simulink model "LKAS_AutoSave_DF_20220407_0926_SW62"  (R2018b)
settings: Solver=FixedStepDiscrete  StartTime=0.0  StopTime=10.0  FixedStep=0.01  RelTol=1e-3
InitFcn:
  | tmpVer = ver('MATLAB');
  | tmpVer = str2num(tmpVer.Version);
  | % -------------------------------------------------------------------
  | %  MATLAB file generated by Simulink.saveVars on 21-Nov-2019 10:06:14
  | %  MATLAB version: 7.13.0.564 (R2011b)
  | % -------------------------------------------------------------------
  | 
  | 
  | SInt16 = Simulink.AliasType;
  | SInt16.Description = 'Num';
  | if (tmpVer > 7.11)
  | 	SInt16.DataScope = 'Auto';
  | end
  | SInt16.HeaderFile = 'Rte_Type.h';
  | SInt16.BaseType = 'int16';
  | 
  | SInt32 = Simulink.AliasType;
  | SInt32.Description = 'Num';
  | if (tmpVer > 7.11)
  | 	SInt32.DataScope = 'Auto';
  | end
  | SInt32.HeaderFile = 'Rte_Type.h';
  | SInt32.BaseType = 'int32';
  | 
  | SInt8 = Simulink.AliasType;
  | SInt8.Description = 'Num';
  | if (tmpVer > 7.11)
  | 	SInt8.DataScope = 'Auto';
  | end
  | SInt8.HeaderFile = 'Rte_Type.h';
  | SInt8.BaseType = 'int8';
  | 
  | T_A_m2_1024_1_u32 = Simulink.NumericType;
  | T_A_m2_1024_1_u32.Description = 'm2 (square meters  (m2))';
  | if (tmpVer > 7.11)
  | 	T_A_m2_1024_1_u32.DataScope = 'Auto';
  | end
  | T_A_m2_1024_1_u32.HeaderFile = 'Rte_Type.h';
  | T_A_m2_1024_1_u32.DataTypeMode = 'Fixed-point: slope and bias scaling';
  | T_A_m2_1024_1_u32.SignednessBool = false;
  | T_A_m2_1024_1_u32.WordLength = 32;
  | T_A_m2_1024_1_u32.FixedExponent = -10;
  | T_A_m2_1024_1_u32.SlopeAdjustmentFactor = 1;
  | T_A_m2_1024_1_u32.Bias = 0;
  | T_A_m2_1024_1_u32.DataTypeOverride = 'Inherit';
  | T_A_m2_1024_1_u32.IsAlias = true;
  | 
  | T_A_m2_65536_1_u16 = Simulink.NumericType;
  | T_A_m2_65536_1_u16.Description = 'm2 (square meters  (m2))';
  | if (tmpVer > 7.11)
  | 	T_A_m2_65536_1_u16.DataScope = 'Auto';
  | end
  | T_A_m2_65536_1_u16.HeaderFile = 'Rte_Type.h';
  | T_A_m2_65536_1_u16.DataTypeMode = 'Fixed-point: slope and bias scaling';
  | T_A_m2_65536_1_u16.SignednessBool = false;
  | T_A_m2_65536_1_u16.WordLength = 16;
  | T_A_m2_65536_1_u16.FixedExponent = -16;
  | T_A_m2_65536_1_u16.SlopeAdjustmentFactor = 1;
  | T_A_m2_65536_1_u16.Bias = 0;
  | T_A_m2_65536_1_u16.DataTypeOverride = 'Inherit';
  | ... (+4664 lines)
StopFcn:
  | clear  T_A_m2_1024_1_u32 T_A_m2_65536_1_u16 T_A_m2_Float32 T_A_mm2_10_1_u16 T_A_mm2_4_1_s16 T_A_mm2_Float32 T_Cnt_Num_10_1_u32 T_Cnt_Num_1_1_s16 T_Cnt_Num_1_1_s32 T_Cnt_Num_1_1_s8 T_Cnt_Num_1_1_u16 T_Cnt_Num_1_1_u32 T_Cnt_Num_1_1_u8 T_E_J_1_1_s32 T_E_J_Float32 T_E_kJ_128_1_s32 T_E_kJ_Float32 T_E_kwh_10_1_u16 T_E_kwh_Float32 T_Epl_kwhpkm_100_1_u16 T_Epl_kwhpkm_Float32 T_F_N_1_1_s16 T_F_N_Float32 T_I_A_1000_1_u16 T_I_A_1048576_1_s32 T_I_A_2048_1_s16 T_I_A_32_1_s16 T_I_A_Float32 T_I_mA_1_1_s16 T_I_mA_32768_128_s16 T_I_mA_Float32 T_J_kgpm2_128_1_u16 T_J_kgpm2_Float32 T_K_NA_1000_1_s16 T_K_NA_100_1_s16 T_K_NA_100_1_u16 T_K_NA_1024_1_s16 T_K_NA_1024_1_u16 T_K_NA_128_1_s16 T_K_NA_128_1_u16 T_K_NA_128_1_u8 T_K_NA_16777216_1_u32 T_K_NA_16_1_s16 T_K_NA_16_1_u16 T_K_NA_16_1_u8 T_K_NA_1_16_u16 T_K_NA_1_1_s16 T_K_NA_1_1_u16 T_K_NA_1_1_u8 T_K_NA_32768_1_s16 T_K_NA_32768_1_u16 T_K_NA_32_1_s8 T_K_NA_4096_1_u16 T_K_NA_4194304_1_s32 T_K_NA_4194304_1_u16 T_K_NA_65536_1_s32 T_K_NA_65536_1_u16 T_K_NA_8192_1_s16 T_K_NA_8_1_s16 T_K_NA_Float32 T_M_Nm_16_1_s16 T_M_Nm_1_1_s16 T_M_Nm_32768_1_s16 T_M_Nm_32_1_s16 T_M_Nm_4_1_s16 T_M_Nm_512_1_s16 T_M_Nm_Float32 T_P_W_1_4_s16 T_P_W_1_8_s16 T_P_W_Float32 T_P_kW_128_1_s16 T_P_kW_1_8_s16 T_P_kW_8_1_s32 T_P_kW_Float32 T_Pct_pct_1024_1_s32 T_Pct_pct_1024_1_u32 T_Pct_pct_10_1_s16 T_Pct_pct_10_1_u32 T_Pct_pct_128_100_s8 T_Pct_pct_1_1_s16 T_Pct_pct_1_4_u8 T_Pct_pct_255_100_u16 T_Pct_pct_255_100_u8 T_Pct_pct_256_1_s16 T_Pct_pct_256_1_u16 T_Pct_pct_65535_100_u16 T_Pct_pct_Float32 T_R_ohm_1024_1_s16 T_R_ohm_32_1_s16 T_R_ohm_Float32 T_TK_K_16_1_s16 T_TK_K_Float32 T_T_degC_10_400_1_u16 T_T_degC_16_1_s16 T_T_degC_1_40_1_u8 T_T_degC_2_80_1_u8 T_T_degC_Float32 T_U_V_1000_1_u16 T_U_V_10_1_u8 T_U_V_200_1_u8 T_U_V_32_1_s16 T_U_V_4096_1_s16 T_U_V_512_1_s16 T_U_V_65535_8_u16 T_U_V_8192_1_u16 T_U_V_Float32 T_U_mV_1_1_s16 T_U_mV_256_20_u16 T_U_mV_Float32 T_V_l_256_1_s16 T_V_l_4096_1_s16 T_V_l_64_1_s16 T_V_l_65535_100_u16 T_V_l_Float32 T_V_ml_128_1_s16 T_V_ml_1_1_s16 T_V_ml_32768_1_s16 T_V_ml_Float32 T_V_ul_32_1_u16 T_V_ul_Float32 T_Vpl_clpkm_512_1_u16 T_Vpl_clpkm_Float32 T_a_kphps_16_1_s16 T_a_kphps_Float32 T_a_mps2_128_1_s16 T_a_mps2_Float32 T_c_MJpkg_256_1_s16 T_c_MJpkg_Float32 T_c_kJpgpK_1024_1_s16 T_c_kJpgpK_Float32 T_c_kJpkgpK_128_1_u16 T_c_kJpkgpK_Float32 T_chrg_Ah_1_1_s16 T_chrg_Ah_1_1_u16 T_chrg_Ah_1_1_u8 T_chrg_Ah_256_1_u16 T_chrg_Ah_4194304_1_s32 T_chrg_Ah_512_1_u16 T_chrg_Ah_8_1_u16 T_chrg_Ah_Float32 T_cmp_NA_100_1_s16 T_cmp_NA_128_1_s16 T_cmp_NA_16_1_s16 T_cmp_NA_32768_1_u16 T_cmp_NA_Float32 T_d2n_rpmps2_4_1_s16 T_d2n_rpmps2_Float32 T_dPct_pctps_16_1_s16 T_dPct_pctps_256_1_s16 T_dPct_pctps_Float32 T_dT_degCps_128_1_s16 T_dT_degCps_Float32 T_dV_lph_1_1_s16 T_dV_lph_Float32 T_dV_lpm_128_1_s16 T_dV_lpm_32_1_s16 T_dV_lpm_Float32 T_dV_lps_1024_1_u16 T_dV_lps_4_1_u16 T_dV_lps_Float32 T_dV_mlps_1024_1_s16 T_dV_mlps_Float32 T_d_BitField16 T_dm_gps_128_1_s16 T_dm_gps_128_1_u16 T_dm_gps_256_1_u16 T_dm_gps_Float32 T_dm_mgps_1_1_s16 T_dm_mgps_Float32 T_dn_rpmps_1_1_s16 T_dn_rpmps_2_1_s16 T_dn_rpmps_Float32 T_dp_Paps_1_1_s16 T_dp_Paps_Float32 T_dp_kPaps_1_1_s16 T_dp_kPaps_8_1_s16 T_dp_kPaps_Float32 T_dphi_degps_128_1_s16 T_dphi_degps_8_1_s16 T_dphi_degps_Float32 T_dr_ps_256_1_s16 T_dr_ps_Float32 T_drho_mgplps_1_2_s16 T_drho_mgplps_Float32 T_e_NA_1_1_u8 T_f_Hz_1_1_u16 T_f_Hz_1_1_u32 T_f_Hz_64_1_u16 T_f_Hz_8_1_s16 T_f_Hz_Float32 T_g_BitField32 T_l_km_16_1_s16 T_l_km_1_1_u16 T_l_km_1_1_u32 T_l_km_Float32 T_l_m_1024_1_s16 T_l_m_16_1_s16 T_l_m_1_1_u32 T_l_m_Float32 T_l_mm_16_1_s16 T_l_mm_1_1_u16 T_l_mm_4096_1_s16 T_l_mm_4_1_u8 T_l_mm_64_1_s16 T_l_mm_Float32 T_m_g_1_1_s16 T_m_g_2048_1_s16 T_m_g_32_1_u16 T_m_g_Float32 T_m_kg_1024_1_s16 T_m_kg_1_1_s16 T_m_kg_1_1_u32 T_m_kg_Float32 T_m_mg_128_1_s16 T_m_mg_32_1_s16 T_m_mg_Float32 T_n_rpm_1_1_s16 T_n_rpm_1_25_u8 T_n_rpm_256_50_u16 T_n_rpm_2_25_u8 T_n_rpm_4_1_u16 T_n_rpm_Float32 T_p_MPa_64_1_s16 T_p_MPa_Float32 T_p_Pa_1_1_s16 T_p_Pa_Float32 T_p_kPa_1_10_u16 T_p_kPa_1_1_s16 T_p_kPa_1_1_u8 T_p_kPa_256_1_u16 T_p_kPa_32_1_u16 T_p_kPa_64_1_s16 T_p_kPa_Float32 T_phi_deg_100_1_s16 T_phi_deg_1024_1_s16 T_phi_deg_128_1_s16 T_phi_deg_1_1_u8 T_phi_deg_256_1_s16 T_phi_deg_2_1_s8 T_phi_deg_32_1_s16 T_phi_deg_512_6_s32 T_phi_deg_Float32 T_phi_rad_2048_1_s16 T_phi_rad_Float32 T_r_NA_1024_1_s16 T_r_NA_1024_1_u16 T_r_NA_16384_1_s16 T_r_NA_16_1_s16 T_r_NA_256_1_s8 T_r_NA_256_1_u16 T_r_NA_32768_1_u16 T_r_NA_32_1_u16 T_r_NA_4096_1_s16 T_r_NA_65535_2_u16 T_r_NA_8192_1_u16 T_r_NA_Float32 T_rho_gpl_8192_1_s16 T_rho_gpl_Float32 T_rho_kgpm3_16_1_s16 T_rho_kgpm3_Float32 T_rho_mgpl_1_1_s16 T_rho_mgpl_64_1_s16 T_rho_mgpl_Float32 T_t_hour_1_1_s16 T_t_hour_Float32 T_t_m_1_1_u16 T_t_m_Float32 T_t_ms_1_1_s16 T_t_ms_1_1_u16 T_t_ms_1_1_u32 T_t_ms_4096_1_s16 T_t_ms_64_1_s16 T_t_ms_Float32 T_t_s_1000_1_s16 T_t_s_100_1_s16 T_t_s_10_1_s16 T_t_s_10_1_u16 T_t_s_1_1_s16 T_t_s_1_1_u16 T_t_s_1_1_u32 T_t_s_Float32 T_t_us_10_1_u32 T_t_us_1_1_s16 T_t_us_1_1_u32 T_t_us_1_4_u16 T_t_us_Float32 T_v_kph_1_1_u8 T_v_kph_64_1_s16 T_v_kph_64_1_u16 T_v_kph_Float32 T_v_mps_256_1_s16 T_v_mps_Float32 T_w_radps_32_1_s16 T_w_radps_Float32 T_y_BitField8 T_y_BitFieldDiagProgress T_y_BitFieldDiagStatus T_y_NA_1_1_u8 SInt16 SInt32 SInt8 T_BOOLEAN UInt16 UInt32 UInt8 s16 s32 s8 u16 u32 u8
model workspace (MAT data in the model file):
  MCOS : class17 (value not decoded)
  MCOS : class17 (value not decoded)
  MCOS : class17 (value not decoded)
  MCOS : class17 (value not decoded)
  MCOS : class17 (value not decoded)
  MCOS : class17 (value not decoded)
  MCOS : class17 (value not decoded)
  MCOS : class17 (value not decoded)
  MCOS : class17 (value not decoded)
  MCOS : class17 (value not decoded)
  MCOS : class17 (value not decoded)
  MCOS : class17 (value not decoded)
  MCOS : class17 (value not decoded)
  MCOS : class17 (value not decoded)
  MCOS : class17 (value not decoded)
  MCOS : class17 (value not decoded)
  MCOS : class17 (value not decoded)
  MCOS : class17 (value not decoded)
  MCOS : class17 (value not decoded)
  MCOS : class17 (value not decoded)
  MCOS : class17 (value not decoded)
  MCOS : class17 (value not decoded)
  MCOS : class17 (value not decoded)
  MCOS : class17 (value not decoded)
  MCOS : class17 (value not decoded)
  MCOS : class17 (value not decoded)
  MCOS : class17 (value not decoded)
  MCOS : class17 (value not decoded)
  MCOS : class17 (value not decoded)
  MCOS : class17 (value not decoded)
  MCOS : class17 (value not decoded)
  MCOS : class17 (value not decoded)
  MCOS : class17 (value not decoded)
  MCOS : class17 (value not decoded)
  MCOS : class17 (value not decoded)
  MCOS : class17 (value not decoded)
  MCOS : class17 (value not decoded)
  MCOS : class17 (value not decoded)
  MCOS : class17 (value not decoded)
  MCOS : class17 (value not decoded)
  MCOS : class17 (value not decoded)
  MCOS : class17 (value not decoded)
  MCOS : class17 (value not decoded)
  MCOS : class17 (value not decoded)
  MCOS : class17 (value not decoded)
  MCOS : class17 (value not decoded)
  MCOS : class17 (value not decoded)
  MCOS : class17 (value not decoded)
  MCOS : class17 (value not decoded)
  MCOS : class17 (value not decoded)
  MCOS : class17 (value not decoded)
  MCOS : class17 (value not decoded)
  MCOS : class17 (value not decoded)
  MCOS : class17 (value not decoded)
  MCOS : class17 (value not decoded)
  MCOS : class17 (value not decoded)
  MCOS : class17 (value not decoded)
  MCOS : class17 (value not decoded)
  MCOS : class17 (value not decoded)
  MCOS : class17 (value not decoded)
  MCOS : class17 (value not decoded)
  MCOS : class17 (value not decoded)
  MCOS : class17 (value not decoded)
  MCOS : class17 (value not decoded)
  MCOS : class17 (value not decoded)
  MCOS : class17 (value not decoded)
  MCOS : class17 (value not decoded)
  MCOS : class17 (value not decoded)
  MCOS : class17 (value not decoded)
  MCOS : class17 (value not decoded)
  MCOS : class17 (value not decoded)
  MCOS : class17 (value not decoded)
  MCOS : class17 (value not decoded)
  MCOS : class17 (value not decoded)
  MCOS : class17 (value not decoded)
  MCOS : class17 (value not decoded)
  MCOS : class17 (value not decoded)
  MCOS : class17 (value not decoded)
  MCOS : class17 (value not decoded)
  MCOS : class17 (value not decoded)
  MCOS : class17 (value not decoded)
  MCOS : class17 (value not decoded)
  MCOS : class17 (value not decoded)
  MCOS : class17 (value not decoded)
  MCOS : class17 (value not decoded)
  MCOS : class17 (value not decoded)
  MCOS : class17 (value not decoded)
  MCOS : class17 (value not decoded)
  MCOS : class17 (value not decoded)
  MCOS : class17 (value not decoded)
  MCOS : class17 (value not decoded)
  MCOS : class17 (value not decoded)
  MCOS : class17 (value not decoded)
  MCOS : class17 (value not decoded)
  MCOS : class17 (value not decoded)
  MCOS : class17 (value not decoded)
  MCOS : class17 (value not decoded)
  MCOS : class17 (value not decoded)
  MCOS : class17 (value not decoded)
  MCOS : class17 (value not decoded)
  MCOS : class17 (value not decoded)
  MCOS : class17 (value not decoded)
  MCOS : class17 (value not decoded)
  MCOS : class17 (value not decoded)
  MCOS : class17 (value not decoded)
  MCOS : class17 (value not decoded)
undefined symbols (not defined in the file): LKA_CarWidth, LKA_SampleTime, LKA_StrRatio_C, LKA_Veh2CamL_C, LKA_Veh2CamW_C, LKA_WhlBaseL_C, LL_CompHdAg_C, LL_CompSWA_C, LL_CrvtPrvwT_C, LL_DesDvt_C, LL_DvtComp_C, LL_DvtPrvwT_C, LL_DvtSpdDet_vDvtSpdMin_C, LL_HandsOff_ExitTime, LL_HandsOff_TextTime, LL_HandsOff_WarnTime, LL_HdAgExT_C, LL_HdAgPrvwT_C, LL_LAccMax_C, LL_LAccRMax_C, LL_LDW_EarliestWarnLine_C, LL_LDW_LatestWarnLine_C, LL_LDWS_SUPPRESS_HEADING, LL_LFClb_TFC_FfCtlRatio_C, LL_LFClb_TFC_KdBalance_C, LL_LFClb_TFC_KdMaxSWA_C, LL_LFClb_TFC_KdV1_C, LL_LFClb_TFC_KdV2_C, LL_LFClb_TFC_KdVehSpdLwr_C, LL_LFClb_TFC_KdVehSpdUpr_C, LL_LFClb_TFC_Ki_C, LL_LFClb_TFC_KiMaxSWA_C, LL_LFClb_TFC_Kp_C, LL_LFClb_TFC_KpKlat_C, LL_LFClb_TFC_KpV1_C, LL_LFClb_TFC_KpV2_C, LL_LFClb_TFC_KpVehSpdLwr_C, LL_LFClb_TFC_KpVehSpdUpr_C, LL_LFClb_TFC_PrvwT_C, LL_LKA_EarliestWarnLine_C, LL_LKA_LatestWarnLine_C, LL_LKAExPrcs_ExitC0Dvt, LL_LKAExPrcs_ExitC0Swt, LL_LKAExPrcs_tiExitDelayTime3, LL_LKAExPrcs_tiExitTime1, LL_LKAExPrcs_tiExitTime2, LL_LKAExPrcs_tiExitTime3, LL_LKAS_OUT_OF_CONTROL_LAT_VEL, LL_LKAS_OUT_OF_CONTROL_TTLC, LL_LKASWASyn_M0, LL_LKASWASyn_M1, LL_LKASWASyn_M2, LL_LKASWASyn_M3D, LL_LKASWASyn_M3K_DT, LL_LKASWASyn_M3K_MSD, LL_LKASWASyn_M4K, LL_LKASWASyn_SWAaddMax, LL_LKASWASyn_T2, LL_LKASWASyn_tiTrqSwaRtTime, LL_LKASWASyn_tiTrqSwaTime ... (+47)
libraries: simulink x234, canmsglib x6, dspstat3 x3, simulink_extras x1
(part 7 of 22)

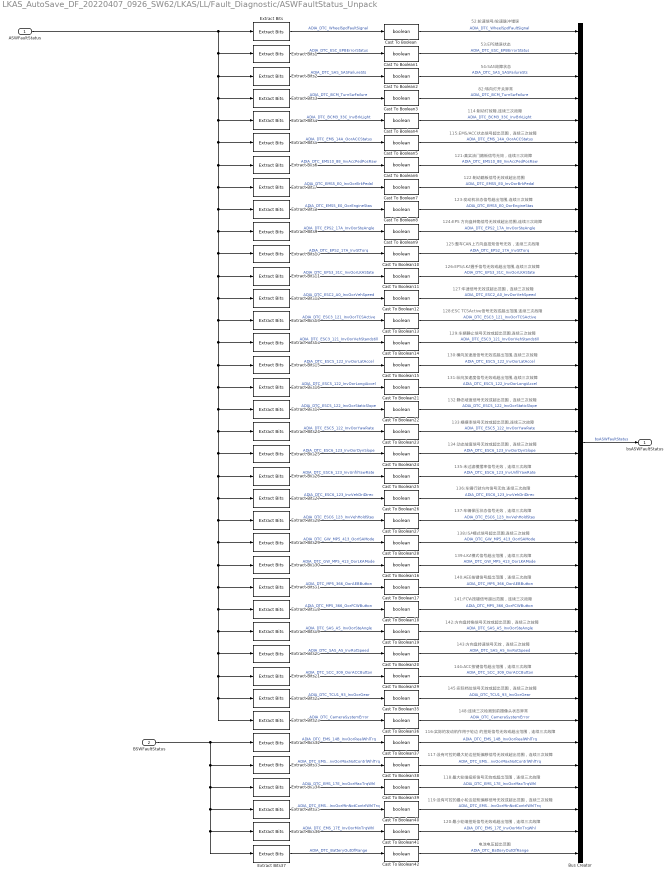
== system LKAS_AutoSave_DF_20220407_0926_SW62/LKAS/LL/Fault_Diagnostic/ASWFaultStatus_Unpack ==
  note: 132:静态坡度信号无效或超出范围，连续三次故障
  note: 133:横摆率信号无效或超出范围,连续三次故障
  note: 135:未过滤横摆率信号无效，连续三次故障
  note: 138:ISA模式信号超出范围,连续三次故障
  note: 136:车辆行驶方向信号无效,连续三次故障
  note: 141:FCW按键信号超出范围，连续三次故障
  note: 127:车速信号无效或超出范围，连续三次故障
  note: 125:整车CAN上方向盘扭矩信号无效，连续三次故障
  note: 126:EPS/LKA握手信号无效或超出范围,连续三次故障
  note: 128:ESC TCSActive信号无效或超出范围,连续三次故障
  note: 140:AEB按键信号超出范围，连续三次故障
  note: 129:车辆静止信号无效或超出范围,连续三次故障
  note: 131:纵向加速度信号无效或超出范围,连续三次故障
  note: 134:动态坡度信号无效或超出范围，连续三次故障
  note: 130:横向加速度信号无效或超出范围,连续三次故障
  note: 52:轮速信号/轮速脉冲错误
  note: 82:转向灯开关异常
  note: 124:EPS 方向盘转角信号无效或超出范围,连续三次故障
  note: 122:制动踏板信号无效或超出范围
  note: 123:发动机状态信号超出范围,连续三次故障
  note: 53:EPB错误状态
  note: 139:LKA模式信号超出范围，连续三次故障
  note: 115:EMS/ACC状态信号超出范围，连续三次故障
  note: 114:制动灯故障,连续三次故障
  note: 137:车辆保压状态信号无效，连续三次故障
  note: 121:真实油门踏板信号无效，连续三次故障
  note: 142:方向盘转角信号无效或超出范围，连续三次故障
  note: 54:SAS故障状态
  note: 145:实际档位信号无效或超出范围，连续三次故障
  note: 144:ACC按键信号超出范围，连续三次故障
  note: 143:方向盘转速信号无效，连续三次故障
  note: 148:连续三次检测到前摄像头状态异常
  note: 电池电压超出范围
  note: 118:最大轮端扭矩信号无效或超出范围，连续三次故障
  note: 119:没有可控的最小轮边扭矩偏移信号无效或超出范围，连续三次故障
  note: 116:实际的发动机作用于轮边 的扭矩信号无效或超出范围，连续三次故障
  note: 120:最小轮端扭矩信号无效或超出范围，连续三次故障
  note: 117:没有可控的最大轮边扭矩偏移信号无效或超出范围，连续三次故障
  ASWFaultStatus : Inport
  BSWFaultStatus : Inport  Port=2
  Bus Creator : BusCreator  Inputs=38
  Cast To Boolean{,1..29,35..42} (38 alike) : DataTypeConversion  OutDataTypeStr=boolean
  Extract Bits : simulink/Logic and Bit Operations/Extract Bits  bitsToExtract=Range of bits  numBits=8  bitIdxRange=0  outScalingMode=Preserve fixed-point scaling
      settings: SourceProductName=Simulink
  Extract Bits1 : simulink/Logic and Bit Operations/Extract Bits  bitsToExtract=Range of bits  numBits=8  bitIdxRange=1  outScalingMode=Treat bit field as an integer
      settings: SourceProductName=Simulink
  Extract Bits10 : simulink/Logic and Bit Operations/Extract Bits  bitsToExtract=Range of bits  numBits=8  bitIdxRange=10  outScalingMode=Treat bit field as an integer
      settings: SourceProductName=Simulink
  Extract Bits11 : simulink/Logic and Bit Operations/Extract Bits  bitsToExtract=Range of bits  numBits=8  bitIdxRange=11  outScalingMode=Treat bit field as an integer
      settings: SourceProductName=Simulink
  Extract Bits12 : simulink/Logic and Bit Operations/Extract Bits  bitsToExtract=Range of bits  numBits=8  bitIdxRange=12  outScalingMode=Treat bit field as an integer
      settings: SourceProductName=Simulink
  Extract Bits13 : simulink/Logic and Bit Operations/Extract Bits  bitsToExtract=Range of bits  numBits=8  bitIdxRange=13  outScalingMode=Treat bit field as an integer
      settings: SourceProductName=Simulink
  Extract Bits14 : simulink/Logic and Bit Operations/Extract Bits  bitsToExtract=Range of bits  numBits=8  bitIdxRange=14  outScalingMode=Treat bit field as an integer
      settings: SourceProductName=Simulink
  Extract Bits15 : simulink/Logic and Bit Operations/Extract Bits  bitsToExtract=Range of bits  numBits=8  bitIdxRange=15  outScalingMode=Treat bit field as an integer
      settings: SourceProductName=Simulink
  Extract Bits16 : simulink/Logic and Bit Operations/Extract Bits  bitsToExtract=Range of bits  numBits=8  bitIdxRange=16  outScalingMode=Treat bit field as an integer
      settings: SourceProductName=Simulink
  Extract Bits17 : simulink/Logic and Bit Operations/Extract Bits  bitsToExtract=Range of bits  numBits=8  bitIdxRange=17  outScalingMode=Treat bit field as an integer
      settings: SourceProductName=Simulink
  Extract Bits18 : simulink/Logic and Bit Operations/Extract Bits  bitsToExtract=Range of bits  numBits=8  bitIdxRange=26  outScalingMode=Treat bit field as an integer
      settings: SourceProductName=Simulink
  Extract Bits19 : simulink/Logic and Bit Operations/Extract Bits  bitsToExtract=Range of bits  numBits=8  bitIdxRange=27  outScalingMode=Treat bit field as an integer
      settings: SourceProductName=Simulink
  Extract Bits2 : simulink/Logic and Bit Operations/Extract Bits  bitsToExtract=Range of bits  numBits=8  bitIdxRange=2  outScalingMode=Treat bit field as an integer
      settings: SourceProductName=Simulink
  Extract Bits20 : simulink/Logic and Bit Operations/Extract Bits  bitsToExtract=Range of bits  numBits=8  bitIdxRange=28  outScalingMode=Treat bit field as an integer
      settings: SourceProductName=Simulink
  Extract Bits21 : simulink/Logic and Bit Operations/Extract Bits  bitsToExtract=Range of bits  numBits=8  bitIdxRange=29  outScalingMode=Treat bit field as an integer
      settings: SourceProductName=Simulink
  Extract Bits22 : simulink/Logic and Bit Operations/Extract Bits  bitsToExtract=Range of bits  numBits=8  bitIdxRange=30  outScalingMode=Treat bit field as an integer
      settings: SourceProductName=Simulink
  Extract Bits23 : simulink/Logic and Bit Operations/Extract Bits  bitsToExtract=Range of bits  numBits=8  bitIdxRange=31  outScalingMode=Treat bit field as an integer
      settings: SourceProductName=Simulink
  Extract Bits24 : simulink/Logic and Bit Operations/Extract Bits  bitsToExtract=Range of bits  numBits=8  bitIdxRange=18  outScalingMode=Treat bit field as an integer
      settings: SourceProductName=Simulink
  Extract Bits25 : simulink/Logic and Bit Operations/Extract Bits  bitsToExtract=Range of bits  numBits=8  bitIdxRange=19  outScalingMode=Treat bit field as an integer
      settings: SourceProductName=Simulink
  Extract Bits26 : simulink/Logic and Bit Operations/Extract Bits  bitsToExtract=Range of bits  numBits=8  bitIdxRange=20  outScalingMode=Treat bit field as an integer
      settings: SourceProductName=Simulink
  Extract Bits27 : simulink/Logic and Bit Operations/Extract Bits  bitsToExtract=Range of bits  numBits=8  bitIdxRange=21  outScalingMode=Treat bit field as an integer
      settings: SourceProductName=Simulink
  Extract Bits28 : simulink/Logic and Bit Operations/Extract Bits  bitsToExtract=Range of bits  numBits=8  bitIdxRange=22  outScalingMode=Treat bit field as an integer
      settings: SourceProductName=Simulink
  Extract Bits29 : simulink/Logic and Bit Operations/Extract Bits  bitsToExtract=Range of bits  numBits=8  bitIdxRange=23  outScalingMode=Treat bit field as an integer
      settings: SourceProductName=Simulink
  Extract Bits3 : simulink/Logic and Bit Operations/Extract Bits  bitsToExtract=Range of bits  numBits=8  bitIdxRange=3  outScalingMode=Treat bit field as an integer
      settings: SourceProductName=Simulink
  Extract Bits30 : simulink/Logic and Bit Operations/Extract Bits  bitsToExtract=Range of bits  numBits=8  bitIdxRange=24  outScalingMode=Treat bit field as an integer
      settings: SourceProductName=Simulink
  Extract Bits31 : simulink/Logic and Bit Operations/Extract Bits  bitsToExtract=Range of bits  numBits=8  bitIdxRange=25  outScalingMode=Treat bit field as an integer
      settings: SourceProductName=Simulink
  Extract Bits32 : simulink/Logic and Bit Operations/Extract Bits  bitsToExtract=Range of bits  numBits=8  bitIdxRange=26  outScalingMode=Treat bit field as an integer
      settings: SourceProductName=Simulink
  Extract Bits33 : simulink/Logic and Bit Operations/Extract Bits  bitsToExtract=Range of bits  numBits=8  bitIdxRange=27  outScalingMode=Treat bit field as an integer
      settings: SourceProductName=Simulink
  Extract Bits34 : simulink/Logic and Bit Operations/Extract Bits  bitsToExtract=Range of bits  numBits=8  bitIdxRange=28  outScalingMode=Treat bit field as an integer
      settings: SourceProductName=Simulink
  Extract Bits35 : simulink/Logic and Bit Operations/Extract Bits  bitsToExtract=Range of bits  numBits=8  bitIdxRange=29  outScalingMode=Treat bit field as an integer
      settings: SourceProductName=Simulink
  Extract Bits36 : simulink/Logic and Bit Operations/Extract Bits  bitsToExtract=Range of bits  numBits=8  bitIdxRange=30  outScalingMode=Treat bit field as an integer
      settings: SourceProductName=Simulink
  Extract Bits37 : simulink/Logic and Bit Operations/Extract Bits  bitsToExtract=Range of bits  numBits=8  bitIdxRange=31  outScalingMode=Treat bit field as an integer
      settings: SourceProductName=Simulink
  Extract Bits4 : simulink/Logic and Bit Operations/Extract Bits  bitsToExtract=Range of bits  numBits=8  bitIdxRange=4  outScalingMode=Treat bit field as an integer
      settings: SourceProductName=Simulink
  Extract Bits5 : simulink/Logic and Bit Operations/Extract Bits  bitsToExtract=Range of bits  numBits=8  bitIdxRange=5  outScalingMode=Treat bit field as an integer
      settings: SourceProductName=Simulink
  Extract Bits6 : simulink/Logic and Bit Operations/Extract Bits  bitsToExtract=Range of bits  numBits=8  bitIdxRange=6  outScalingMode=Treat bit field as an integer
      settings: SourceProductName=Simulink
  Extract Bits7 : simulink/Logic and Bit Operations/Extract Bits  bitsToExtract=Range of bits  numBits=8  bitIdxRange=7  outScalingMode=Treat bit field as an integer
      settings: SourceProductName=Simulink
  Extract Bits8 : simulink/Logic and Bit Operations/Extract Bits  bitsToExtract=Range of bits  numBits=8  bitIdxRange=8  outScalingMode=Treat bit field as an integer
      settings: SourceProductName=Simulink
  Extract Bits9 : simulink/Logic and Bit Operations/Extract Bits  bitsToExtract=Range of bits  numBits=8  bitIdxRange=9  outScalingMode=Treat bit field as an integer
      settings: SourceProductName=Simulink
  bsASWFaultStatus : Outport
  wires:
  ASWFaultStatus/1 -> Extract Bits/1, Extract Bits1/1, Extract Bits2/1, Extract Bits3/1, Extract Bits4/1, Extract Bits5/1, Extract Bits6/1, Extract Bits7/1, Extract Bits8/1, Extract Bits9/1, Extract Bits10/1, Extract Bits11/1, Extract Bits12/1, Extract Bits13/1, Extract Bits14/1, Extract Bits15/1, Extract Bits16/1, Extract Bits17/1, Extract Bits24/1, Extract Bits25/1, Extract Bits26/1, Extract Bits27/1, Extract Bits28/1, Extract Bits29/1, Extract Bits30/1, Extract Bits31/1, Extract Bits18/1, Extract Bits19/1, Extract Bits20/1, Extract Bits21/1, Extract Bits22/1, Extract Bits23/1
  Cast To Boolean35/1 -> Bus Creator/31  "ADIA_DTC_TCU1_93_InvOorGear"
  Cast To Boolean2/1 -> Bus Creator/3  "ADIA_DTC_SAS_SASFailureSts"
  Cast To Boolean1/1 -> Bus Creator/2  "ADIA_DTC_ESC_EPBErrorStatus"
  Cast To Boolean13/1 -> Bus Creator/14  "ADIA_DTC_ESC3_121_InvOorTCSActive"
  Cast To Boolean19/1 -> Bus Creator/28  "ADIA_DTC_SAS_A5_InvOorSteAngle"
  Cast To Boolean26/1 -> Bus Creator/22  "ADIA_DTC_ESC6_123_InvVehDriDirec"
  Cast To Boolean5/1 -> Bus Creator/6  "ADIA_DTC_EMS_14A_OorACCStatus"
  Cast To Boolean14/1 -> Bus Creator/15  "ADIA_DTC_ESC3_121_InvOorVehStandstill"
  Cast To Boolean10/1 -> Bus Creator/11  "ADIA_DTC_EPS2_17A_InvStTorq"
  Cast To Boolean11/1 -> Bus Creator/12  "ADIA_DTC_EPS3_31C_InvOorLKAState"
  Cast To Boolean12/1 -> Bus Creator/13  "ADIA_DTC_ESC2_A0_InvOorVehSpeed"
  Cast To Boolean28/1 -> Bus Creator/24  "ADIA_DTC_GW_MP5_413_OorISAMode"
  Cast To Boolean18/1 -> Bus Creator/27  "ADIA_DTC_MP5_366_OorFCWButton"
  Cast To Boolean22/1 -> Bus Creator/18  "ADIA_DTC_ESC5_122_InvOorStaticSlope"
  Cast To Boolean/1 -> Bus Creator/1  "ADIA_DTC_WheelSpdFaultSignal"
  Cast To Boolean23/1 -> Bus Creator/19  "ADIA_DTC_ESC5_122_InvOorYawRate"
  Bus Creator/1 -> bsASWFaultStatus/1  "bsASWFaultStatus"
  Cast To Boolean15/1 -> Bus Creator/16  "ADIA_DTC_ESC5_122_InvOorLatAccel"
  Cast To Boolean8/1 -> Bus Creator/9  "ADIA_DTC_EMS5_E0_OorEngineStas"
  Cast To Boolean27/1 -> Bus Creator/23  "ADIA_DTC_ESC6_123_InvVehHoldStas"
  Cast To Boolean17/1 -> Bus Creator/26  "ADIA_DTC_MP5_366_OorAEBButton"
  Cast To Boolean4/1 -> Bus Creator/5  "ADIA_DTC_BCM3_33C_InvBrkLight"
  Cast To Boolean3/1 -> Bus Creator/4  "ADIA_DTC_BCM_TurnSwFailure"
  Cast To Boolean7/1 -> Bus Creator/8  "ADIA_DTC_EMS5_E0_InvOorBrkPedal"
  Cast To Boolean6/1 -> Bus Creator/7  "ADIA_DTC_EMS10_88_InvAccPedPosRaw"
  Cast To Boolean9/1 -> Bus Creator/10  "ADIA_DTC_EPS2_17A_InvOorSteAngle"
  Cast To Boolean21/1 -> Bus Creator/17  "ADIA_DTC_ESC5_122_InvOorLongiAccel"
  Cast To Boolean24/1 -> Bus Creator/20  "ADIA_DTC_ESC6_123_InvOorDynSlope"
  Cast To Boolean25/1 -> Bus Creator/21  "ADIA_DTC_ESC6_123_InvUnfilYawRate"
  Cast To Boolean20/1 -> Bus Creator/29  "ADIA_DTC_SAS_A5_InvRotSpeed"
  Cast To Boolean16/1 -> Bus Creator/25  "ADIA_DTC_GW_MP5_413_OorLKAMode"
  Cast To Boolean29/1 -> Bus Creator/30  "ADIA_DTC_SCC_309_OorACCButton"
  Cast To Boolean36/1 -> Bus Creator/32  "ADIA_DTC_CameraSystemError"
  Cast To Boolean42/1 -> Bus Creator/38  "ADIA_DTC_BatteryOutOfRange"
  Cast To Boolean41/1 -> Bus Creator/37  "ADIA_DTC_EMS_17E_InvOorMinTrqWhl"
  Cast To Boolean40/1 -> Bus Creator/36  "ADIA_DTC_EMS_17E_InvOorMinNotContrlWhlTrq"
  Cast To Boolean38/1 -> Bus Creator/34  "ADIA_DTC_EMS_17E_InvOorMaxNotContrlWhlTrq"
  Cast To Boolean39/1 -> Bus Creator/35  "ADIA_DTC_EMS_17E_InvOorMaxTrqWhl"
  BSWFaultStatus/1 -> Extract Bits32/1, Extract Bits33/1, Extract Bits34/1, Extract Bits35/1, Extract Bits36/1, Extract Bits37/1
  Cast To Boolean37/1 -> Bus Creator/33  "ADIA_DTC_EMS_14B_InvOorRealWhlTrq"
  Extract Bits/1 -> Cast To Boolean/1  "ADIA_DTC_WheelSpdFaultSignal"
  Extract Bits1/1 -> Cast To Boolean1/1  "ADIA_DTC_ESC_EPBErrorStatus"
  Extract Bits2/1 -> Cast To Boolean2/1  "ADIA_DTC_SAS_SASFailureSts"
  Extract Bits3/1 -> Cast To Boolean3/1  "ADIA_DTC_BCM_TurnSwFailure"
  Extract Bits4/1 -> Cast To Boolean4/1  "ADIA_DTC_BCM3_33C_InvBrkLight"
  Extract Bits5/1 -> Cast To Boolean5/1  "ADIA_DTC_EMS_14A_OorACCStatus"
  Extract Bits6/1 -> Cast To Boolean6/1  "ADIA_DTC_EMS10_88_InvAccPedPosRaw"
  Extract Bits7/1 -> Cast To Boolean7/1  "ADIA_DTC_EMS5_E0_InvOorBrkPedal"
  Extract Bits8/1 -> Cast To Boolean8/1  "ADIA_DTC_EMS5_E0_OorEngineStas"
  Extract Bits9/1 -> Cast To Boolean9/1  "ADIA_DTC_EPS2_17A_InvOorSteAngle"
  Extract Bits10/1 -> Cast To Boolean10/1  "ADIA_DTC_EPS2_17A_InvStTorq"
  Extract Bits11/1 -> Cast To Boolean11/1  "ADIA_DTC_EPS3_31C_InvOorLKAState"
  Extract Bits12/1 -> Cast To Boolean12/1  "ADIA_DTC_ESC2_A0_InvOorVehSpeed"
  Extract Bits13/1 -> Cast To Boolean13/1  "ADIA_DTC_ESC3_121_InvOorTCSActive"
  Extract Bits14/1 -> Cast To Boolean14/1  "ADIA_DTC_ESC3_121_InvOorVehStandstill"
  Extract Bits15/1 -> Cast To Boolean15/1  "ADIA_DTC_ESC5_122_InvOorLatAccel"
  Extract Bits16/1 -> Cast To Boolean21/1  "ADIA_DTC_ESC5_122_InvOorLongiAccel"
  Extract Bits17/1 -> Cast To Boolean22/1  "ADIA_DTC_ESC5_122_InvOorStaticSlope"
  Extract Bits24/1 -> Cast To Boolean23/1  "ADIA_DTC_ESC5_122_InvOorYawRate"
  Extract Bits25/1 -> Cast To Boolean24/1  "ADIA_DTC_ESC6_123_InvOorDynSlope"
  Extract Bits26/1 -> Cast To Boolean25/1  "ADIA_DTC_ESC6_123_InvUnfilYawRate"
  Extract Bits27/1 -> Cast To Boolean26/1  "ADIA_DTC_ESC6_123_InvVehDriDirec"
  Extract Bits28/1 -> Cast To Boolean27/1  "ADIA_DTC_ESC6_123_InvVehHoldStas"
  Extract Bits29/1 -> Cast To Boolean28/1  "ADIA_DTC_GW_MP5_413_OorISAMode"
  Extract Bits30/1 -> Cast To Boolean16/1  "ADIA_DTC_GW_MP5_413_OorLKAMode"
  Extract Bits31/1 -> Cast To Boolean17/1  "ADIA_DTC_MP5_366_OorAEBButton"
  Extract Bits18/1 -> Cast To Boolean18/1  "ADIA_DTC_MP5_366_OorFCWButton"
  Extract Bits19/1 -> Cast To Boolean19/1  "ADIA_DTC_SAS_A5_InvOorSteAngle"
  Extract Bits20/1 -> Cast To Boolean20/1  "ADIA_DTC_SAS_A5_InvRotSpeed"
  Extract Bits21/1 -> Cast To Boolean29/1  "ADIA_DTC_SCC_309_OorACCButton"
  Extract Bits22/1 -> Cast To Boolean35/1  "ADIA_DTC_TCU1_93_InvOorGear"
  Extract Bits23/1 -> Cast To Boolean36/1  "ADIA_DTC_CameraSystemError"
  Extract Bits32/1 -> Cast To Boolean37/1  "ADIA_DTC_EMS_14B_InvOorRealWhlTrq"
  Extract Bits33/1 -> Cast To Boolean38/1  "ADIA_DTC_EMS_17E_InvOorMaxNotContrlWhlTrq"
  Extract Bits34/1 -> Cast To Boolean39/1  "ADIA_DTC_EMS_17E_InvOorMaxTrqWhl"
  Extract Bits35/1 -> Cast To Boolean40/1  "ADIA_DTC_EMS_17E_InvOorMinNotContrlWhlTrq"
  Extract Bits36/1 -> Cast To Boolean41/1  "ADIA_DTC_EMS_17E_InvOorMinTrqWhl"
  Extract Bits37/1 -> Cast To Boolean42/1  "ADIA_DTC_BatteryOutOfRange"

== system LKAS_AutoSave_DF_20220407_0926_SW62/LKAS/LL/Fault_Diagnostic/BSWFaultStatus_Unpack ==
  note: EPS节点通信丢失
  note: TCU节点通信丢失
  note: TBox节点通信丢失
  note: MP5节点通信丢失
  note: IC节点通信丢失
  note: EMS节点通信丢失
  note: ESC节点通信丢失
  note: SAS节点通信丢失
  note: BCM节点通信丢失
  note: ACU节点通信丢失
  note: EPB节点通信丢失
  note: 前雷达内部故障
  note: 角雷达故障
  BSWFaultStatus : Inport
  Bus Creator : BusCreator  Inputs=13
  Cast To Boolean{,1..12} (13 alike) : DataTypeConversion  OutDataTypeStr=boolean
  Extract Bits : simulink/Logic and Bit Operations/Extract Bits  bitsToExtract=Range of bits  numBits=8  bitIdxRange=0  outScalingMode=Treat bit field as an integer
      settings: SourceProductName=Simulink
  Extract Bits1 : simulink/Logic and Bit Operations/Extract Bits  bitsToExtract=Range of bits  numBits=8  bitIdxRange=1  outScalingMode=Treat bit field as an integer
      settings: SourceProductName=Simulink
  Extract Bits10 : simulink/Logic and Bit Operations/Extract Bits  bitsToExtract=Range of bits  numBits=8  bitIdxRange=10  outScalingMode=Treat bit field as an integer
      settings: SourceProductName=Simulink
  Extract Bits16 : simulink/Logic and Bit Operations/Extract Bits  bitsToExtract=Range of bits  numBits=8  bitIdxRange=16  outScalingMode=Treat bit field as an integer
      settings: SourceProductName=Simulink
  Extract Bits17 : simulink/Logic and Bit Operations/Extract Bits  bitsToExtract=Range of bits  numBits=8  bitIdxRange=17  outScalingMode=Treat bit field as an integer
      settings: SourceProductName=Simulink
  Extract Bits2 : simulink/Logic and Bit Operations/Extract Bits  bitsToExtract=Range of bits  numBits=8  bitIdxRange=2  outScalingMode=Treat bit field as an integer
      settings: SourceProductName=Simulink
  Extract Bits3 : simulink/Logic and Bit Operations/Extract Bits  bitsToExtract=Range of bits  numBits=8  bitIdxRange=3  outScalingMode=Treat bit field as an integer
      settings: SourceProductName=Simulink
  Extract Bits4 : simulink/Logic and Bit Operations/Extract Bits  bitsToExtract=Range of bits  numBits=8  bitIdxRange=4  outScalingMode=Treat bit field as an integer
      settings: SourceProductName=Simulink
  Extract Bits5 : simulink/Logic and Bit Operations/Extract Bits  bitsToExtract=Range of bits  numBits=8  bitIdxRange=5  outScalingMode=Treat bit field as an integer
      settings: SourceProductName=Simulink
  Extract Bits6 : simulink/Logic and Bit Operations/Extract Bits  bitsToExtract=Range of bits  numBits=8  bitIdxRange=6  outScalingMode=Treat bit field as an integer
      settings: SourceProductName=Simulink
  Extract Bits7 : simulink/Logic and Bit Operations/Extract Bits  bitsToExtract=Range of bits  numBits=8  bitIdxRange=7  outScalingMode=Treat bit field as an integer
      settings: SourceProductName=Simulink
  Extract Bits8 : simulink/Logic and Bit Operations/Extract Bits  bitsToExtract=Range of bits  numBits=8  bitIdxRange=8  outScalingMode=Treat bit field as an integer
      settings: SourceProductName=Simulink
  Extract Bits9 : simulink/Logic and Bit Operations/Extract Bits  bitsToExtract=Range of bits  numBits=8  bitIdxRange=9  outScalingMode=Treat bit field as an integer
      settings: SourceProductName=Simulink
  bsBSWFaultStatus : Outport
  wires:
  Cast To Boolean11/1 -> Bus Creator/12  "ADIA_Inner_FRadar_FaultState"
  Cast To Boolean9/1 -> Bus Creator/10  "ADIAve_e_Node_TCU_Validity"
  Cast To Boolean6/1 -> Bus Creator/7  "ADIAve_e_Node_IC_Validity"
  Cast To Boolean7/1 -> Bus Creator/8  "ADIAve_e_Node_TBOX_Validity"
  Cast To Boolean3/1 -> Bus Creator/4  "ADIAve_e_Node_IBCM_Validity"
  Cast To Boolean4/1 -> Bus Creator/5  "ADIAve_e_Node_SAS_Validity"
  Cast To Boolean8/1 -> Bus Creator/9  "ADIAve_e_Node_MP5_Validity"
  Bus Creator/1 -> bsBSWFaultStatus/1  "bsBSWFaultStatus"
  Cast To Boolean/1 -> Bus Creator/1  "ADIAve_e_Node_ACU_Validity"
  Cast To Boolean12/1 -> Bus Creator/13  "ADIAve_d_sen_sta_Corner_radar"
  Cast To Boolean10/1 -> Bus Creator/11  "ADIAve_e_Node_EPB_Validity"
  Cast To Boolean5/1 -> Bus Creator/6  "ADIAve_e_Node_EMS_Validity"
  Cast To Boolean1/1 -> Bus Creator/2  "ADIAve_e_Node_EPS_Validity"
  Cast To Boolean2/1 -> Bus Creator/3  "ADIAve_e_Node_ESC_Validity"
  BSWFaultStatus/1 -> Extract Bits/1, Extract Bits1/1, Extract Bits2/1, Extract Bits3/1, Extract Bits4/1, Extract Bits5/1, Extract Bits6/1, Extract Bits7/1, Extract Bits8/1, Extract Bits9/1, Extract Bits10/1, Extract Bits17/1, Extract Bits16/1
  Extract Bits/1 -> Cast To Boolean/1  "ADIAve_e_Node_ACU_Validity"
  Extract Bits1/1 -> Cast To Boolean1/1  "ADIAve_e_Node_EPS_Validity"
  Extract Bits2/1 -> Cast To Boolean2/1  "ADIAve_e_Node_ESC_Validity"
  Extract Bits3/1 -> Cast To Boolean3/1  "ADIAve_e_Node_IBCM_Validity"
  Extract Bits4/1 -> Cast To Boolean4/1  "ADIAve_e_Node_SAS_Validity"
  Extract Bits5/1 -> Cast To Boolean5/1  "ADIAve_e_Node_EMS_Validity"
  Extract Bits6/1 -> Cast To Boolean6/1  "ADIAve_e_Node_IC_Validity"
  Extract Bits7/1 -> Cast To Boolean7/1  "ADIAve_e_Node_TBOX_Validity"
  Extract Bits8/1 -> Cast To Boolean8/1  "ADIAve_e_Node_MP5_Validity"
  Extract Bits9/1 -> Cast To Boolean9/1  "ADIAve_e_Node_TCU_Validity"
  Extract Bits10/1 -> Cast To Boolean10/1  "ADIAve_e_Node_EPB_Validity"
  Extract Bits16/1 -> Cast To Boolean11/1  "ADIA_Inner_FRadar_FaultState"
  Extract Bits17/1 -> Cast To Boolean12/1  "ADIAve_d_sen_sta_Corner_radar"

== system LKAS_AutoSave_DF_20220407_0926_SW62/LKAS/LL/Fault_Diagnostic/FuncFaultStatus_Unpack ==
  note: ob_ADIA_SpareDataCheck
  FuncFaultStatus : Inport
  Bus Creator : BusCreator  Inputs=16
  Extract Bits : simulink/Logic and Bit Operations/Extract Bits  bitsToExtract=Range of bits  numBits=8  bitIdxRange=0  outScalingMode=Treat bit field as an integer
      settings: SourceProductName=Simulink
  Extract Bits1 : simulink/Logic and Bit Operations/Extract Bits  bitsToExtract=Range of bits  numBits=8  bitIdxRange=1  outScalingMode=Treat bit field as an integer
      settings: SourceProductName=Simulink
  Extract Bits10 : simulink/Logic and Bit Operations/Extract Bits  bitsToExtract=Range of bits  numBits=8  bitIdxRange=10  outScalingMode=Treat bit field as an integer
      settings: SourceProductName=Simulink
  Extract Bits11 : simulink/Logic and Bit Operations/Extract Bits  bitsToExtract=Range of bits  numBits=8  bitIdxRange=11  outScalingMode=Treat bit field as an integer
      settings: SourceProductName=Simulink
  Extract Bits12 : simulink/Logic and Bit Operations/Extract Bits  bitsToExtract=Range of bits  numBits=8  bitIdxRange=12  outScalingMode=Treat bit field as an integer
      settings: SourceProductName=Simulink
  Extract Bits13 : simulink/Logic and Bit Operations/Extract Bits  bitsToExtract=Range of bits  numBits=8  bitIdxRange=13  outScalingMode=Treat bit field as an integer
      settings: SourceProductName=Simulink
  Extract Bits14 : simulink/Logic and Bit Operations/Extract Bits  bitsToExtract=Range of bits  numBits=8  bitIdxRange=14  outScalingMode=Treat bit field as an integer
      settings: SourceProductName=Simulink
  Extract Bits15 : simulink/Logic and Bit Operations/Extract Bits  bitsToExtract=Range of bits  numBits=8  bitIdxRange=15  outScalingMode=Treat bit field as an integer
      settings: SourceProductName=Simulink
  Extract Bits2 : simulink/Logic and Bit Operations/Extract Bits  bitsToExtract=Range of bits  numBits=8  bitIdxRange=2  outScalingMode=Treat bit field as an integer
      settings: SourceProductName=Simulink
  Extract Bits3 : simulink/Logic and Bit Operations/Extract Bits  bitsToExtract=Range of bits  numBits=8  bitIdxRange=3  outScalingMode=Treat bit field as an integer
      settings: SourceProductName=Simulink
  Extract Bits4 : simulink/Logic and Bit Operations/Extract Bits  bitsToExtract=Range of bits  numBits=8  bitIdxRange=4  outScalingMode=Treat bit field as an integer
      settings: SourceProductName=Simulink
  Extract Bits5 : simulink/Logic and Bit Operations/Extract Bits  bitsToExtract=Range of bits  numBits=8  bitIdxRange=5  outScalingMode=Treat bit field as an integer
      settings: SourceProductName=Simulink
  Extract Bits6 : simulink/Logic and Bit Operations/Extract Bits  bitsToExtract=Range of bits  numBits=8  bitIdxRange=6  outScalingMode=Treat bit field as an integer
      settings: SourceProductName=Simulink
  Extract Bits7 : simulink/Logic and Bit Operations/Extract Bits  bitsToExtract=Range of bits  numBits=8  bitIdxRange=7  outScalingMode=Treat bit field as an integer
      settings: SourceProductName=Simulink
  Extract Bits8 : simulink/Logic and Bit Operations/Extract Bits  bitsToExtract=Range of bits  numBits=8  bitIdxRange=8  outScalingMode=Treat bit field as an integer
      settings: SourceProductName=Simulink
  Extract Bits9 : simulink/Logic and Bit Operations/Extract Bits  bitsToExtract=Range of bits  numBits=8  bitIdxRange=9  outScalingMode=Treat bit field as an integer
      settings: SourceProductName=Simulink
  bsFuncFaultStatus : Outport
  wires:
  FuncFaultStatus/1 -> Extract Bits/1, Extract Bits1/1, Extract Bits2/1, Extract Bits3/1, Extract Bits4/1, Extract Bits5/1, Extract Bits6/1, Extract Bits7/1, Extract Bits8/1, Extract Bits9/1, Extract Bits10/1, Extract Bits11/1, Extract Bits12/1, Extract Bits13/1, Extract Bits14/1, Extract Bits15/1
  Extract Bits2/1 -> Bus Creator/3
  Extract Bits1/1 -> Bus Creator/2
  Extract Bits13/1 -> Bus Creator/14  "ob_DTC_ACC_Displacement_Safety_Violation"
  Extract Bits5/1 -> Bus Creator/6
  Extract Bits14/1 -> Bus Creator/15  "ob_DTC_ACC_HoldConfirm_Safety_Violation"
  Extract Bits10/1 -> Bus Creator/11
  Extract Bits11/1 -> Bus Creator/12  "ob_DTC_ACC_Accel_Decel_Safety_Violation"
  Extract Bits12/1 -> Bus Creator/13  "ob_DTC_ACC_Mixed_Mode_Conflict"
  Extract Bits/1 -> Bus Creator/1
  Bus Creator/1 -> bsFuncFaultStatus/1  "bsFuncFaultStatus"
  Extract Bits15/1 -> Bus Creator/16  "ob_DTC_AEB_Safety_Violation"
  Extract Bits8/1 -> Bus Creator/9  "ob_ADIA_SpareDataCheck"
  Extract Bits4/1 -> Bus Creator/5
  Extract Bits3/1 -> Bus Creator/4
  Extract Bits7/1 -> Bus Creator/8
  Extract Bits6/1 -> Bus Creator/7
  Extract Bits9/1 -> Bus Creator/10

== system LKAS_AutoSave_DF_20220407_0926_SW62/LKAS/LL/Human Machine Interface (HMI)/Subsystem ==
  LDW_State : Inport
  LKA_State : Inport  Port=2
  bsEPSInfo : Inport  Port=3
  LKA_SampleTime : Inport  Port=4
  LL_HandsOff_TextTime : Inport  Port=5
  LL_HandsOff_WarnTime : Inport  Port=6
  LL_RlsDet_tiTrqChkT_DISABLE : Inport  Port=7
  LL_RlsDet_tiTrqChkT_EPS_DISABLE : Inport  Port=8
  Abs : Abs
  Bus Selector2 : BusSelector  OutputSignals=EPS_LKA_State,EPS_SW_Trq
  Compare{1..2,4,7} (4 alike) : simulink/Logic and Bit Operations/Compare To Constant  relop===  const=3  OutDataTypeStr=boolean
  Compare3 : simulink/Logic and Bit Operations/Compare To Constant  relop===  const=1  OutDataTypeStr=boolean
  Compare5 : simulink/Logic and Bit Operations/Compare To Constant  relop===  const=4  OutDataTypeStr=boolean
  Compare6 : simulink/Logic and Bit Operations/Compare To Constant  relop===  const=5  OutDataTypeStr=boolean
  Compare8 : simulink/Logic and Bit Operations/Compare To Constant  relop===  const=4  OutDataTypeStr=boolean
  Compare9 : simulink/Logic and Bit Operations/Compare To Constant  relop===  const=5  OutDataTypeStr=boolean
  Logical Operator1 : Logic  Operator=OR  AllPortsSameDT=off  OutDataTypeStr=boolean
  Logical Operator2 : Logic  Inputs=3  AllPortsSameDT=off  OutDataTypeStr=boolean
  Logical Operator3 : Logic  Operator=OR  Inputs=6  AllPortsSameDT=off  OutDataTypeStr=boolean
  Relational Operator : RelationalOperator  Operator=<=  OutDataTypeStr=boolean  RndMeth=Nearest
  Sum Condition1 : Subsystem  TreatAsAtomicUnit=on
  Sum Condition2 : Subsystem  TreatAsAtomicUnit=on
  Switch : Switch  Criteria=u2 > Threshold
  HandsOff2_Warn : Outport
  HandsOff1_Text : Outport  Port=2
  wires:
  Sum Condition1/1(Out) -> HandsOff1_Text/1
  Bus Selector2/1 -> Compare3/1, Compare2/1, Compare1/1  "<EPS_LKA_State>"
  LL_RlsDet_tiTrqChkT_EPS_DISABLE/1 -> Switch/1
  bsEPSInfo/1 -> Bus Selector2/1
  Switch/1 -> Relational Operator/2
  Compare1/1 -> Switch/2
  Logical Operator2/1 -> Sum Condition2/Enable, Sum Condition1/Enable
  Logical Operator3/1 -> Logical Operator2/1
  LL_RlsDet_tiTrqChkT_DISABLE/1 -> Switch/3
  Relational Operator/1 -> Logical Operator2/3
  Sum Condition2/1(Out) -> HandsOff2_Warn/1
  LDW_State/1 -> Compare4/1, Compare6/1, Compare5/1
  Compare4/1 -> Logical Operator3/3
  Compare5/1 -> Logical Operator3/2
  Compare6/1 -> Logical Operator3/1
  Abs/1 -> Relational Operator/1
  LKA_State/1 -> Compare9/1, Compare8/1, Compare7/1
  Compare9/1 -> Logical Operator3/4
  Compare8/1 -> Logical Operator3/5
  Compare7/1 -> Logical Operator3/6
  Compare2/1 -> Logical Operator1/1
  Compare3/1 -> Logical Operator1/2
  Logical Operator1/1 -> Logical Operator2/2
  [LKA_SampleTime] -> Sum Condition1/1(SampleTime), Sum Condition2/1(SampleTime)
  LL_HandsOff_TextTime/1 -> Sum Condition1/2(Sum)
  LL_HandsOff_WarnTime/1 -> Sum Condition2/2(Sum)
  Bus Selector2/2 -> Abs/1  "<EPS_SW_Trq>"
  LKA_SampleTime/1 -> [LKA_SampleTime]

== system LKAS_AutoSave_DF_20220407_0926_SW62/LKAS/LL/LL Inputs Mapping/bsBCMInfo ==
  bsBCMInfoIn : Inport
  Bus Creator1 : BusCreator  Inputs=3
  Bus Selector1 : BusSelector  OutputSignals=BCM_Double_Light,BCM_Left_Light,BCM_Right_Light,BCM_LeftTurn_Switch,BCM_RightTurn_Switch
  Compare To Constant : simulink/Logic and Bit Operations/Compare To Constant  relop===  const=1  OutDataTypeStr=boolean
  Compare To Constant1 : simulink/Logic and Bit Operations/Compare To Constant  relop===  const=1  OutDataTypeStr=boolean
  Logical Operator : Logic  Operator=OR  AllPortsSameDT=off  OutDataTypeStr=boolean
  Logical Operator1 : Logic  Operator=OR  AllPortsSameDT=off  OutDataTypeStr=boolean
  bsBCMInfoOut : Outport
  wires:
  Bus Selector1/3 -> Logical Operator1/1  "<BCM_Right_Light>"
  Bus Selector1/2 -> Logical Operator/1  "<BCM_Left_Light>"
  Bus Creator1/1 -> bsBCMInfoOut/1
  Bus Selector1/1 -> Bus Creator1/1  "<BCM_Double_Light>"
  bsBCMInfoIn/1 -> Bus Selector1/1
  Bus Selector1/4 -> Compare To Constant/1  "<BCM_LeftTurn_Switch>"
  Bus Selector1/5 -> Compare To Constant1/1  "<BCM_RightTurn_Switch>"
  Compare To Constant/1 -> Logical Operator/2
  Compare To Constant1/1 -> Logical Operator1/2
  Logical Operator/1 -> Bus Creator1/2  "BCM_Left_Light"
  Logical Operator1/1 -> Bus Creator1/3  "BCM_Right_Light"

== system LKAS_AutoSave_DF_20220407_0926_SW62/LKAS/LL/LL Inputs Mapping/bsEPSInfo ==
  bsEPSInfoIn : Inport
  Bus Creator4 : BusCreator  Inputs=11
  Bus Selector1 : BusSelector  OutputSignals=EPS_LKA_State,EPS_SW_Trq,EPS_Trq_State,SAS_Clb_State,SAS_Trim_State,SWS_Failure_Status,EPS_TrqLim_State,EPS_LKA_Current,EPS_SWHold_State,EPS_Driver_Override,EPS_ESA_State
  bsEPSInfoOut : Outport
  wires:
  Bus Selector1/9 -> Bus Creator4/9  "<EPS_SWHold_State>"
  Bus Selector1/8 -> Bus Creator4/8  "<EPS_LKA_Current>"
  Bus Selector1/7 -> Bus Creator4/7  "<EPS_TrqLim_State>"
  Bus Selector1/5 -> Bus Creator4/5  "<SAS_Trim_State>"
  Bus Selector1/4 -> Bus Creator4/4  "<SAS_Clb_State>"
  Bus Selector1/3 -> Bus Creator4/3  "<EPS_Trq_State>"
  Bus Creator4/1 -> bsEPSInfoOut/1
  Bus Selector1/1 -> Bus Creator4/1  "<EPS_LKA_State>"
  Bus Selector1/2 -> Bus Creator4/2  "<EPS_SW_Trq>"
  bsEPSInfoIn/1 -> Bus Selector1/1
  Bus Selector1/6 -> Bus Creator4/6  "<SWS_Failure_Status>"
  Bus Selector1/10 -> Bus Creator4/10  "<EPS_Driver_Override>"
  Bus Selector1/11 -> Bus Creator4/11  "<EPS_ESA_State>"

== system LKAS_AutoSave_DF_20220407_0926_SW62/LKAS/LL/LL Inputs Mapping/bsLaneInfo ==
  bsLLClb : Inport
  bsLaneInfoIn : Inport  Port=2
  Bus Creator : BusCreator  Inputs=5
  Bus Selector1 : BusSelector  OutputSignals=bsFusL0Info,bsFusR0Info,bsFusL1Info,bsFusR1Info,bsFusLrgInfo,bsFusRrgInfo,Fusion_AdditionalInf
  LaneSelect : Subsystem
  "LanesReconstruct " : Subsystem
  bsLaneInfoOut : Outport
  wires:
  Bus Creator/1 -> bsLaneInfoOut/1
  Bus Selector1/4 -> LaneSelect/4(bsFusR1Info)  "<bsFusR1Info>"
  Bus Selector1/3 -> LaneSelect/3(bsFusL1Info)  "<bsFusL1Info>"
  Bus Selector1/2 -> LaneSelect/2(bsFusR0Info)  "<bsFusR0Info>"
  Bus Selector1/1 -> LaneSelect/1(bsFusL0Info)  "<bsFusL0Info>"
  LaneSelect/4(bsR1Info) -> "LanesReconstruct "/5(bsR1Info)
  LaneSelect/3(bsL1Info) -> "LanesReconstruct "/4(bsL1Info)
  LaneSelect/2(bsR0Info) -> "LanesReconstruct "/3(bsR0Info)
  LaneSelect/1(bsL0Info) -> "LanesReconstruct "/2(bsL0Info)
  "LanesReconstruct "/4(bsR1InfoR) -> Bus Creator/4  "bsR1Info"
  "LanesReconstruct "/3(bsL1InfoR) -> Bus Creator/3  "bsL1Info"
  "LanesReconstruct "/2(bsR0InfoR) -> Bus Creator/2  "bsR0Info"
  "LanesReconstruct "/1(bsL0InfoR) -> Bus Creator/1  "bsL0Info"
  Bus Selector1/7 -> Bus Creator/5  "<Fusion_AdditionalInf>"
  bsLaneInfoIn/1 -> Bus Selector1/1
  bsLLClb/1 -> "LanesReconstruct "/1(bsLLClb)
  Bus Selector1/5 -> LaneSelect/5(bsFusLrgInfo)  "<bsFusLrgInfo>"
  Bus Selector1/6 -> LaneSelect/6(bsFusRrgInfo)  "<bsFusRrgInfo>"
  LaneSelect/5(bsLrgInfo) -> "LanesReconstruct "/6(bsLrgInfo)
  LaneSelect/6(bsRrgInfo) -> "LanesReconstruct "/7(bsRrgInfo)

== system LKAS_AutoSave_DF_20220407_0926_SW62/LKAS/LL/LL Inputs Mapping/bsMP5Info ==
  note: LDW_Warn_Mode
      | 0: 声音
      | 1: 振动
      | 2: 声音+振动
  note: LkaFcnConf
      | 0: OFF
      | 1: LDW-声音
      | 2: LDW-振动
      | 3: LDW-声音+振动
      | 4: LKA-声音
      | 5: LKA-振动
      | 6: LKA-声音+振动
      | 7: LDW-声音-ICA
      | 8: LDW-振动-ICA
      | 9: LDW-声音+振动-ICA
      | 10: LKA-声音-ICA
      | 11: LKA-振动-ICA
      | 12: LKA-声音+振动-ICA
  note: LKA_Mode
      | 0: LDW
      | 1: LKA
      | 2: ~
  note: LKA_Mode
      | 0: off
      | 1: LDW
      | 2: LKA
  note: ELK_Mode
      | 0: off
      | 1: LDW
      | 2: ~
      | 3: ELK
  bsMP5InfoIn : Inport
  Bus Creator : BusCreator  Inputs=6
  Bus Selector1 : BusSelector  OutputSignals=LkaFcnConf,LKA_Main_Switch,LKA_Mode,LDW_Warn_Mode,APA_AutoPark_WorkSt,MP5_Work_State
  Cast To Boolean : DataTypeConversion  OutDataTypeStr=boolean
  MATLAB Function : MATLAB Function  TreatAsAtomicUnit=on
  bsMP5InfoOut : Outport
  wires:
  bsMP5InfoIn/1 -> Bus Selector1/1
  Bus Selector1/5 -> Bus Creator/5  "<APA_AutoPark_WorkSt>"
  Bus Selector1/6 -> Bus Creator/6  "<MP5_Work_State>"
  Bus Creator/1 -> bsMP5InfoOut/1
  Bus Selector1/3 -> MATLAB Function/3(LKA_Mode_In)  "<LKA_Mode>"
  Bus Selector1/4 -> MATLAB Function/4(LDW_Warn_Mode_In)  "<LDW_Warn_Mode>"
  MATLAB Function/3(LKA_Mode) -> Bus Creator/3  "LKA_Mode"
  MATLAB Function/4(LDW_Warn_Mode) -> Bus Creator/4  "LDW_Warn_Mode"
  MATLAB Function/1(LKA_Main_Switch) -> Bus Creator/1  "LKA_Main_Switch"
  Bus Selector1/1 -> MATLAB Function/1(LkaFcnConf)  "<LkaFcnConf>"
  Bus Selector1/2 -> Cast To Boolean/1  "<LKA_Main_Switch>"
  MATLAB Function/2(LKA_Switch) -> Bus Creator/2  "LKA_Switch"
  Cast To Boolean/1 -> MATLAB Function/2(LKA_Main_Switch_In)

== system LKAS_AutoSave_DF_20220407_0926_SW62/LKAS/LL/LL Inputs Mapping/bsPTState ==
  bsPTStateIn : Inport
  Bus Creator3 : BusCreator  Inputs=3
  Bus Selector1 : BusSelector  OutputSignals=AccPedal_Pos,TCU_ActualGear,TCU_Available
  Constant1 : Constant  Value=0  OutDataTypeStr=uint8
  Constant3 : Constant  Value=3  OutDataTypeStr=uint8
  Multiport Switch : MultiPortSwitch  DataPortOrder=Zero-based contiguous  Inputs=11  zeroidx=on
  bsPTStateOut : Outport
  wires:
  Bus Creator3/1 -> bsPTStateOut/1
  Bus Selector1/1 -> Bus Creator3/1  "<AccPedal_Pos>"
  bsPTStateIn/1 -> Bus Selector1/1
  Multiport Switch/1 -> Bus Creator3/2  "TCU_ActualGear"
  Constant3/1 -> Multiport Switch/11, Multiport Switch/10, Multiport Switch/9, Multiport Switch/6, Multiport Switch/5, Multiport Switch/4, Multiport Switch/3
  Bus Selector1/2 -> Multiport Switch/1  "<TCU_ActualGear>"
  Constant1/1 -> Multiport Switch/12, Multiport Switch/8, Multiport Switch/7, Multiport Switch/2
  Bus Selector1/3 -> Bus Creator3/3  "<TCU_Available>"

== system LKAS_AutoSave_DF_20220407_0926_SW62/LKAS/LL/LL Inputs Mapping/bsSWAInfo ==
  bsSWAInfoIn : Inport
  Bus Creator : BusCreator  Inputs=4
  Bus Selector1 : BusSelector  OutputSignals=EPS_SteeringAngle_Flag,EPS_SteeringAngle,SW_Angle,SW_Angle_Speed
  Gain : Gain
  bsSWAInfoOut : Outport
  wires:
  Bus Creator/1 -> bsSWAInfoOut/1
  Bus Selector1/4 -> Bus Creator/4  "<SW_Angle_Speed>"
  Gain/1 -> Bus Creator/3  "SW_Angle"
  bsSWAInfoIn/1 -> Bus Selector1/1
  Bus Selector1/2 -> Bus Creator/2, Gain/1  "<EPS_SteeringAngle>"
  Bus Selector1/1 -> Bus Creator/1  "<EPS_SteeringAngle_Flag>"
